simulink model "W03_2_vrx_nav"  (R2024b)
settings: Solver=FixedStepDiscrete  StartTime=0.0  StopTime=T_end  FixedStep=Ts  RelTol=1e-3
values from neighbouring files (symbols this model uses):
  alt0 = 1.183941401541233    (= 1.18394140154)    [W03_setup.m]
  animate = 1    [W03_setup.m]
  lat0 = -33.72276870341191    (= -33.7227687034)    [W03_setup.m]
  lon0 = 150.67399057896623    (= 150.673990579)    [W03_setup.m]
  Ts = 0.05    [W03_setup.m]
libraries: ros2lib x2
settings Model: Creator=admin  LastModifiedBy=admin

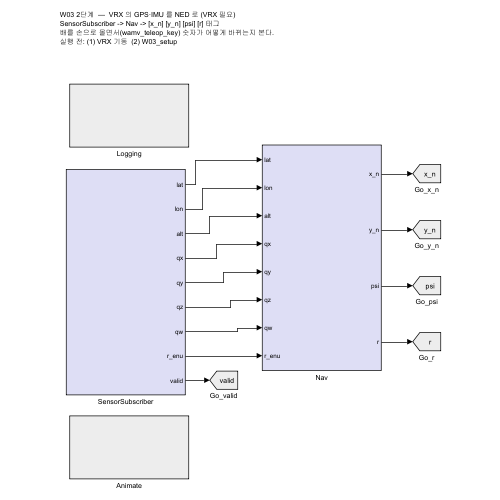
[thumbnail: Simulink's stored preview of the top-level diagram]
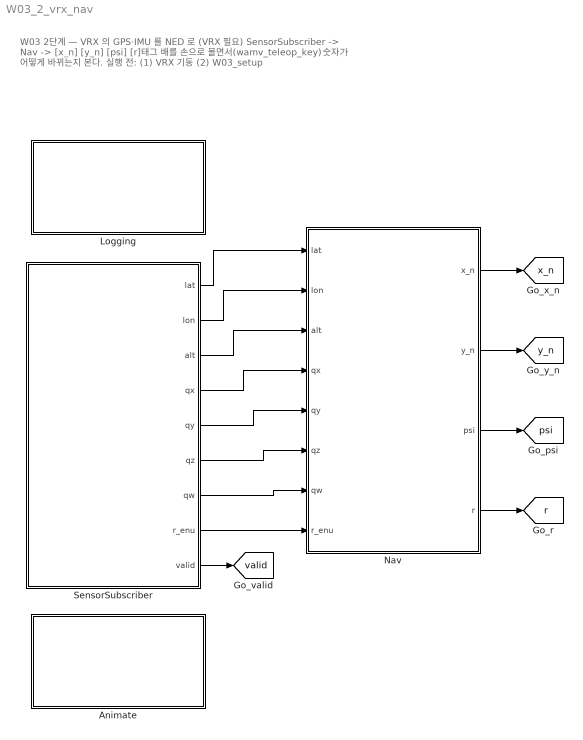
== system W03_2_vrx_nav ==
  note: W03 2단계  —  VRX 의 GPS·IMU 를 NED 로 (VRX 필요)
      | SensorSubscriber -> Nav -> [x_n] [y_n] [psi] [r] 태그
      | 배를 손으로 몰면서(wamv_teleop_key) 숫자가 어떻게 바뀌는지 본다.
      | 실행 전: (1) VRX 기동  (2) W03_setup
  Animate : Subsystem
  Logging : Subsystem
  Nav : Subsystem
  SensorSubscriber : Subsystem
  tag scope: psi=global, r=global, valid=global, x_n=global, y_n=global
  wires:
  SensorSubscriber/1(lat) -> Nav/1(lat)
  SensorSubscriber/3(alt) -> Nav/3(alt)
  SensorSubscriber/7(qw) -> Nav/7(qw)
  SensorSubscriber/2(lon) -> Nav/2(lon)
  SensorSubscriber/6(qz) -> Nav/6(qz)
  SensorSubscriber/5(qy) -> Nav/5(qy)
  SensorSubscriber/4(qx) -> Nav/4(qx)
  SensorSubscriber/8(r_enu) -> Nav/8(r_enu)
  Nav/1(x_n) -> [x_n]
  Nav/2(y_n) -> [y_n]
  Nav/3(psi) -> [psi]
  Nav/4(r) -> [r]
  SensorSubscriber/9(valid) -> [valid]

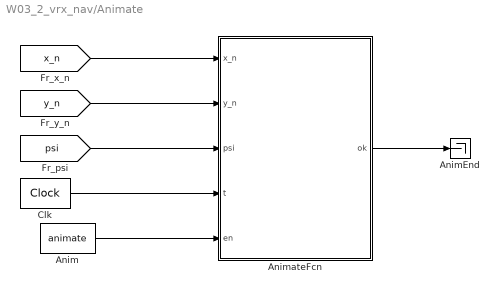
== system W03_2_vrx_nav/Animate ==
  Anim : Constant  Value=animate
  AnimEnd : Terminator
  AnimateFcn : MATLAB Function  TreatAsAtomicUnit=on
  Clk : DigitalClock  SampleTime=Ts
  wires:
  [x_n] -> AnimateFcn/1(x_n)
  [y_n] -> AnimateFcn/2(y_n)
  [psi] -> AnimateFcn/3(psi)
  Clk/1 -> AnimateFcn/4(t)
  Anim/1 -> AnimateFcn/5(en)
  AnimateFcn/1(ok) -> AnimEnd/1

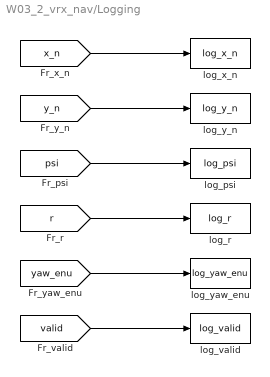
== system W03_2_vrx_nav/Logging ==
  log_psi : ToWorkspace  VariableName=log_psi  SaveFormat=Timeseries  SampleTime=Ts
  log_r : ToWorkspace  VariableName=log_r  SaveFormat=Timeseries  SampleTime=Ts
  log_valid : ToWorkspace  VariableName=log_valid  SaveFormat=Timeseries  SampleTime=Ts
  log_x_n : ToWorkspace  VariableName=log_x_n  SaveFormat=Timeseries  SampleTime=Ts
  log_y_n : ToWorkspace  VariableName=log_y_n  SaveFormat=Timeseries  SampleTime=Ts
  log_yaw_enu : ToWorkspace  VariableName=log_yaw_enu  SaveFormat=Timeseries  SampleTime=Ts
  wires:
  [x_n] -> log_x_n/1
  [y_n] -> log_y_n/1
  [psi] -> log_psi/1
  [r] -> log_r/1
  [yaw_enu] -> log_yaw_enu/1
  [valid] -> log_valid/1

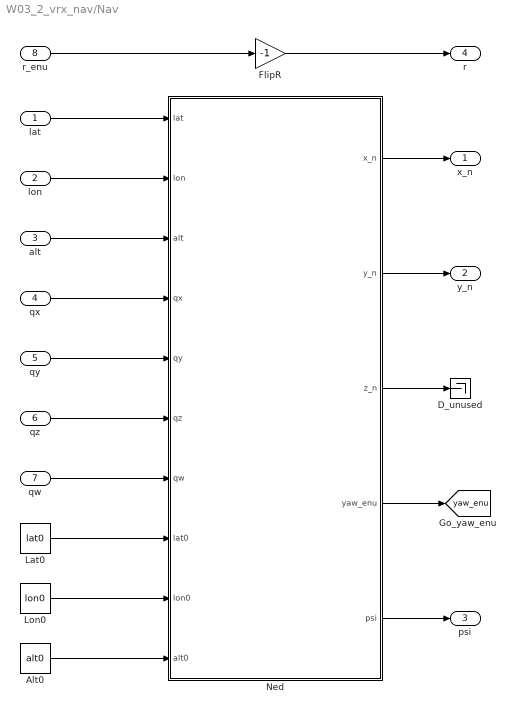
== system W03_2_vrx_nav/Nav ==
  lat : Inport
  lon : Inport  Port=2
  alt : Inport  Port=3
  qx : Inport  Port=4
  qy : Inport  Port=5
  qz : Inport  Port=6
  qw : Inport  Port=7
  r_enu : Inport  Port=8
  Alt0 : Constant  Value=alt0
  D_unused : Terminator
  FlipR : Gain  Gain=-1
  Lat0 : Constant  Value=lat0
  Lon0 : Constant  Value=lon0
  Ned : MATLAB Function  TreatAsAtomicUnit=on
  x_n : Outport
  y_n : Outport  Port=2
  psi : Outport  Port=3
  r : Outport  Port=4
  tag scope: yaw_enu=global
  wires:
  Alt0/1 -> Ned/10(alt0)
  qy/1 -> Ned/5(qy)
  qw/1 -> Ned/7(qw)
  r_enu/1 -> FlipR/1
  qz/1 -> Ned/6(qz)
  lat/1 -> Ned/1(lat)
  lon/1 -> Ned/2(lon)
  qx/1 -> Ned/4(qx)
  alt/1 -> Ned/3(alt)
  FlipR/1 -> r/1
  Lat0/1 -> Ned/8(lat0)
  Lon0/1 -> Ned/9(lon0)
  Ned/5(psi) -> psi/1
  Ned/1(x_n) -> x_n/1
  Ned/2(y_n) -> y_n/1
  Ned/3(z_n) -> D_unused/1
  Ned/4(yaw_enu) -> [yaw_enu]

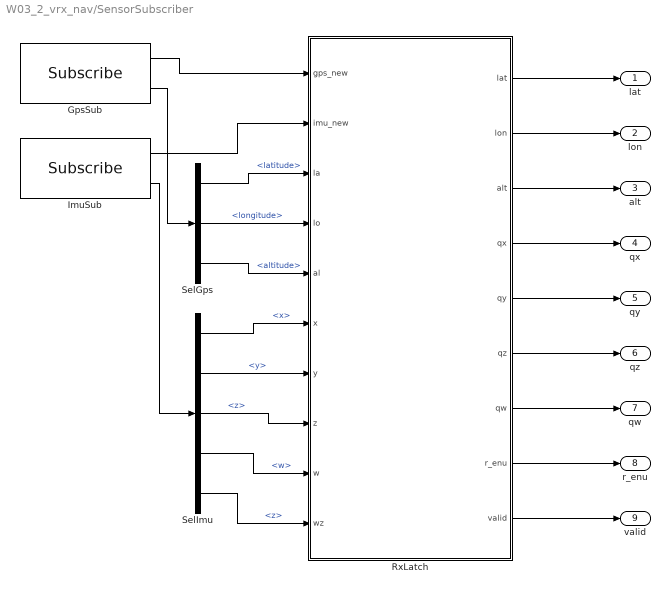
== system W03_2_vrx_nav/SensorSubscriber ==
  GpsSub : ros2lib/Subscribe  topicSource=Specify your own  topic=/wamv/sensors/gps/gps/fix  messageType=sensor_msgs/NavSatFix  sampleTime=Ts  QOSHistory=Keep last  QOSDepth=1  QOSReliability=Reliable  QOSDurability=Volatile  QOSDeadline=Inf  QOSLifespan=Inf  QOSLiveliness=Automatic  QOSLeaseDuration=Inf  QOSAvoidROSNamespaceConventions=off
  ImuSub : ros2lib/Subscribe  topicSource=Specify your own  topic=/wamv/sensors/imu/imu/data  messageType=sensor_msgs/Imu  sampleTime=Ts  QOSHistory=Keep last  QOSDepth=1  QOSReliability=Reliable  QOSDurability=Volatile  QOSDeadline=Inf  QOSLifespan=Inf  QOSLiveliness=Automatic  QOSLeaseDuration=Inf  QOSAvoidROSNamespaceConventions=off
  RxLatch : MATLAB Function  TreatAsAtomicUnit=on
  SelGps : BusSelector  OutputSignals=latitude,longitude,altitude
  SelImu : BusSelector  OutputSignals=orientation.x,orientation.y,orientation.z,orientation.w,angular_velocity.z
  lat : Outport
  lon : Outport  Port=2
  alt : Outport  Port=3
  qx : Outport  Port=4
  qy : Outport  Port=5
  qz : Outport  Port=6
  qw : Outport  Port=7
  r_enu : Outport  Port=8
  valid : Outport  Port=9
  wires:
  GpsSub/1 -> RxLatch/1(gps_new)
  ImuSub/2 -> SelImu/1
  ImuSub/1 -> RxLatch/2(imu_new)
  GpsSub/2 -> SelGps/1
  SelGps/2 -> RxLatch/4(lo)  "<longitude>"
  SelImu/1 -> RxLatch/6(x)  "<x>"
  SelGps/3 -> RxLatch/5(al)  "<altitude>"
  SelGps/1 -> RxLatch/3(la)  "<latitude>"
  SelImu/2 -> RxLatch/7(y)  "<y>"
  SelImu/3 -> RxLatch/8(z)  "<z>"
  SelImu/4 -> RxLatch/9(w)  "<w>"
  SelImu/5 -> RxLatch/10(wz)  "<z>"
  RxLatch/9(valid) -> valid/1
  RxLatch/5(qy) -> qy/1
  RxLatch/1(lat) -> lat/1
  RxLatch/2(lon) -> lon/1
  RxLatch/7(qw) -> qw/1
  RxLatch/3(alt) -> alt/1
  RxLatch/8(r_enu) -> r_enu/1
  RxLatch/4(qx) -> qx/1
  RxLatch/6(qz) -> qz/1

== matlab function W03_2_vrx_nav/Nav/Ned ==
  data: lat input; x_n output; lon input; alt input; qx input; qy input; qz input; qw input; lat0 input; lon0 input; alt0 input; y_n output; z_n output; yaw_enu output; psi output
function [x_n, y_n, z_n, yaw_enu, psi] = Ned(lat, lon, alt, qx, qy, qz, qw, lat0, lon0, alt0)
%#codegen
% ENU(ROS/Gazebo) -> NED(ship control). W03 section 1-5, 1-6.
%   position : flat-earth approximation around (lat0, lon0)
%   heading  : quaternion (ROS order x,y,z,w) -> yaw_ENU -> psi_NED

a  = 6378137.0;              % WGS84 semi-major axis [m]
e2 = 6.69437999014e-3;       % WGS84 first eccentricity squared

lat0r = lat0*pi/180;
s2    = sin(lat0r)^2;
Rm    = a*(1 - e2) / (1 - e2*s2)^1.5;      % meridian radius
Rn    = a / sqrt(1 - e2*s2);               % prime vertical radius

x_n =  (lat - lat0)*pi/180 * Rm;           % north [m]
y_n =  (lon - lon0)*pi/180 * Rn*cos(lat0r);% east  [m]
z_n = -(alt - alt0);                       % down  [m]

% yaw about ENU z (up). ROS quaternion order is (x, y, z, w).
yaw_enu = atan2(2*(qw*qz + qx*qy), 1 - 2*(qy*qy + qz*qz));
p   = pi/2 - yaw_enu;                      % NED heading
psi = atan2(sin(p), cos(p));               % wrap to [-pi, pi)

== matlab function W03_2_vrx_nav/SensorSubscriber/RxLatch ==
  data: gps_new input; lat output; imu_new input; la input; lo input; al input; x input; y input; z input; w input; wz input; lon output; alt output; qx output; qy output; qz output; qw output; r_enu output; valid output
function [lat, lon, alt, qx, qy, qz, qw, r_enu, valid] = RxLatch(gps_new, imu_new, la, lo, al, x, y, z, w, wz)
%#codegen
% Subscribe blocks output an all-zero message before the first one arrives.
% Latitude 0 / longitude 0 is a real place (Gulf of Guinea), so the value
% cannot be used to tell "no data yet" apart. Latch the IsNew flags instead.
persistent seen_gps seen_imu
if isempty(seen_gps), seen_gps = false; seen_imu = false; end
if gps_new, seen_gps = true; end
if imu_new, seen_imu = true; end

lat = la;  lon = lo;  alt = al;
qx  = x;   qy  = y;   qz  = z;  qw = w;
r_enu = wz;
valid = double(seen_gps && seen_imu);

== matlab function W03_2_vrx_nav/Animate/AnimateFcn ==
  data: x_n input; ok output; y_n input; psi input; t input; en input
function ok = AnimateFcn(x_n, y_n, psi, t, en)
%#codegen
coder.extrinsic('W03_animate');
ok = 1;
if en > 0.5
    W03_animate(x_n, y_n, psi, t);
end
